simulink model "LPF"  (R2018b)
settings: Solver=FixedStepAuto  StartTime=0.0  StopTime=10.0  FixedStep=0.01  RelTol=1e-3
settings Model: Creator=kshat  LastModifiedBy=m152069
settings OptimizationCC: DefaultParameterBehavior=Inlined  UseDivisionForNetSlopeComputation=on  UseFloatMulNetSlope=on  InlineInvariantSignals=on  PassReuseOutputArgsAs=Individual arguments  ZeroExternalMemoryAtStartup=off  ZeroInternalMemoryAtStartup=off  NoFixptDivByZeroProtection=on  EfficientFloat2IntCast=on  LifeSpan=1  OptimizeBlockOrder=speed  DifferentSizesBufferReuse=on
settings DebuggingCC: ParameterTunabilityLossMsg=error  LibraryContextMissingDiagnostic=none
settings HardwareCC: ProdBitPerPointer=32  ProdBitPerSizeT=32  ProdBitPerPtrDiffT=32  ProdLargestAtomicInteger=Long  ProdWordSize=32  ProdLongLongMode=on  ProdHWDeviceType=ARM Compatible->ARM 9
settings SFSimCC: SimUseLocalCustomCode=off  MATLABDynamicMemAlloc=off
settings RTWCC: SystemTargetFile=ert.tlc  TemplateMakefile=ert_default_tmf  GenerateReport=on  RTWUseLocalCustomCode=off  IncludeHyperlinkInReport=on  LaunchReport=on  TargetLang=C++  GenerateTraceInfo=on  GenerateTraceReport=on  GenerateTraceReportSl=on  GenerateTraceReportSf=on  GenerateTraceReportEml=on
settings CodeAppCC: ForceParamTrailComments=on  IgnoreCustomStorageClasses=off  OperatorAnnotations=on  SimulinkDataObjDesc=on  SFDataObjDesc=on  CustomSymbolStrGlobalVar=rt$N$M  CustomSymbolStrType=$N$M  CustomSymbolStrFcn=$N$M$F  CustomSymbolStrMacro=$N$M  InsertBlockDesc=on
settings ERTTargetCC: TargetLangStandard=C++03 (ISO)  GenerateSampleERTMain=on  IncludeMdlTerminateFcn=off  CombineSignalStateStructs=on  SuppressErrorStatus=on  SupportAbsoluteTime=off  MultiInstanceERTCode=on  CodeInterfacePackaging=C++ class  SupportComplex=off  InlinedParameterPlacement=NonHierarchical  RootIOFormat=Structure reference  ERTCustomFileTemplate=example_file_process.tlc  ERTFilePackagingFormat=CompactWithDataFile

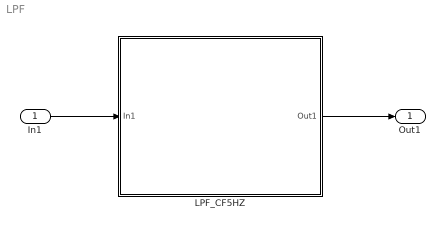
== system LPF ==
  In1 : Inport
  LPF_CF5HZ : Subsystem  TreatAsAtomicUnit=on
  Out1 : Outport
  wires:
  In1/1 -> LPF_CF5HZ/1(In1)
  LPF_CF5HZ/1(Out1) -> Out1/1

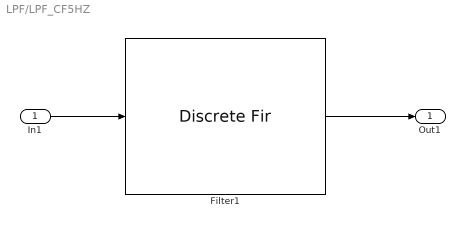
== system LPF/LPF_CF5HZ ==
  In1 : Inport
  Filter1 : DiscreteFir  Tag=BlockMethodSubSystem  Coefficients=[0.00456087975259436649 -0.00181663348337506698 -0.00182639167312229913 -0.00199240452484161909 -0.0022381839856466107 -0.00249538444821011682 -0.00270291804299660487 -0.00280510532316929299 -0.00275500046501173232 -0.00251725175002385972 -0.00207315439026600117 -0.00141750753523047271 -0.000561391998989817904 0.000458416599144693124 0.00159556605357077854 0.00277983075809552175 0.00393173632424987166 0.00496174280142075777 0.00577693930094417153 0.00628786667645815384 0.00641458332502943453 0.00609591379136947917 0.00529250440078157022 0.00399595645083018237 0.00223159266608123543 5.8977961717700188e-05 -0.00242347014642375382 -0.00508538676123084909 -0.00776561106152528786 -0.0102807076974250691 -0.0124333183047034557 -0.0140219846326852648 -0.0148549422334195956 -0.0147567357170871622 -0.013587180750866415 -0.0112447114986979572 -0.00767891398850178725 -0.00289744108858680733 0.00303400468245583086 0.00998796737258814821 0.0177796041025792204 0.0261724948139632797 0.034889006274162998 0.0436249336662691278 0.0520490400094173813 0.0598553759775868402 0.0667176897962276083 0.0723712769066276046 0.0765895410024716866 0.0791945864731981031 0.0800755787018147397 0.0791945864731981031 0.0765895410024716866 0.0723712769066276046 0.0667176897962276083 0.0598553759775868402 0.0520490400094173813 0.0436249336662691278 0.034889006274162998 0.0261724948139632797 0.0177796041025792204 0.00998796737258814821 0.00303400468245583086 -0.00289744108858680733 -0.00767891398850178725 -0.0112447114986979572 -0.013587180750866415 -0.0147567357170871622 -0.0148549422334195956 -0.0140219846326852648 -0.0124333183047034557 -0.0102807076974250691 -0.00776561106152528786 -0.00508538676123084909 -0.00242347014642375382 5.8977961717700188e-05 0.00223159266608123543 0.00399595645083018237 0.00529250440078157022 0.00609591379136947917 0.00641458332502943453 0.00628786667645815384 0.00577693930094417153 0.00496174280142075777 0.00393173632424987166 0.00277983075809552175 0.00159556605357077854 0.000458416599144693124 -0.000561391998989817904 -0.00141750753523047271 -0.00207315439026600117 -0.00251725175002385972 -0.00275500046501173232 -0.00280510532316929299 -0.00270291804299660487 -0.00249538444821011682 -0.0022381839856466107 -0.00199240452484161909 -0.00182639167312229913 -0.00181663348337506698 0.00456087975259436649]  InputProcessing=Columns as channels (frame based)
  Out1 : Outport
  wires:
  Filter1/1 -> Out1/1
  In1/1 -> Filter1/1
